simulink model "model_ekf"  (R2016a)
settings: Solver=VariableStepAuto  StartTime=0.0  StopTime=50  FixedStep=T  RelTol=1e-3
undefined symbols (not defined in the file): C, g, I, K, k1, k2, Ki, l, m, Q, sigbuilder_block, T_sens, Ts
libraries: aerolibutil x2
settings Model: Creator=Patrick  LastModifiedBy=Patrick

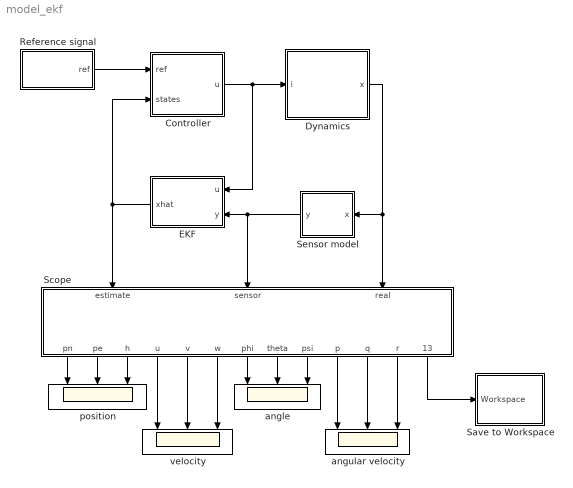
== system model_ekf ==
  Controller : Subsystem
  Dynamics : Subsystem
  EKF : Subsystem
  Reference signal : Subsystem
  Save to Workspace : Subsystem
  Scope : Subsystem
  Sensor model : Subsystem
  angle : Scope  NumInputPorts=3
  angular velocity : Scope  NumInputPorts=3
  position : Scope  NumInputPorts=3
  velocity : Scope  NumInputPorts=3
  wires:
  Sensor model/1(y) -> Scope/2(sensor), EKF/2(y)
  Reference signal/1(ref) -> Controller/1(ref)
  EKF/1(xhat) -> Scope/1(estimate), Controller/2(states)
  Dynamics/1(x) -> Scope/3(real), Sensor model/1(x)
  Controller/1(u) -> EKF/1(u), Dynamics/1(i)
  Scope/5(v) -> velocity/2
  Scope/6(w) -> velocity/3
  Scope/8(theta) -> angle/2
  Scope/9(psi) -> angle/3
  Scope/11(q) -> angular velocity/2
  Scope/10(p) -> angular velocity/1
  Scope/12(r) -> angular velocity/3
  Scope/1(pn) -> position/1
  Scope/2(pe) -> position/2
  Scope/3(h) -> position/3
  Scope/4(u) -> velocity/1
  Scope/7(phi) -> angle/1
  Scope/13(Workspace) -> Save to Workspace/1(Workspace)

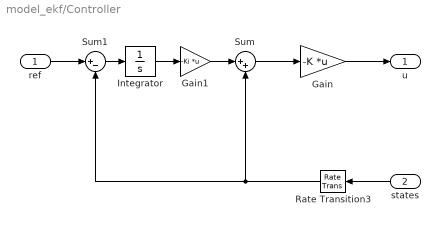
== system model_ekf/Controller ==
  ref : Inport
  states : Inport  Port=2
  Gain : Gain  Gain=-K  Multiplication=Matrix(K*u)
  Gain1 : Gain  Gain=-Ki  Multiplication=Matrix(K*u)
  Integrator : Integrator  InitialCondition=[0;0;0;0;0;0;0;0;0;0;0;0]
  Rate Transition3 : RateTransition  OutPortSampleTime=T
  Sum : Sum  Inputs=|++
  Sum1 : Sum  Inputs=|+-
  u : Outport
  wires:
  Gain1/1 -> Sum/1
  ref/1 -> Sum1/1
  Sum1/1 -> Integrator/1
  Integrator/1 -> Gain1/1
  states/1 -> Rate Transition3/1
  Sum/1 -> Gain/1
  Gain/1 -> u/1
  Rate Transition3/1 -> Sum1/2, Sum/2

== system model_ekf/Dynamics ==
  i : Inport
  Dynamics : Subsystem
  Mux : Mux
  x : Outport
  wires:
  Mux/1 -> x/1
  i/1 -> Dynamics/1(delta)
  Dynamics/1(pn pe h) -> Mux/1
  Dynamics/2(u v w) -> Mux/2
  Dynamics/3(phi theta psi) -> Mux/3
  Dynamics/4(p q r) -> Mux/4

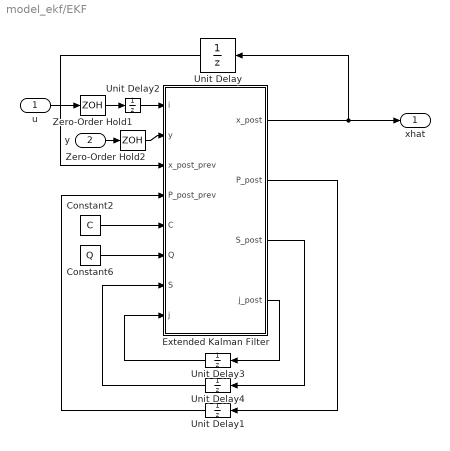
== system model_ekf/EKF ==
  u : Inport
  y : Inport  Port=2
  Constant2 : Constant  Value=C
  Constant6 : Constant  Value=Q
  Extended Kalman Filter : MATLAB Function  TreatAsAtomicUnit=on
  Unit Delay : UnitDelay  InitialCondition=[0;0;0;0;0;0;0;0;0;0;0;0]  SampleTime=Ts
  Unit Delay1 : UnitDelay  InitialCondition=zeros(12,12)  SampleTime=Ts
  Unit Delay2 : UnitDelay  InitialCondition=[0;0;0;0]  SampleTime=Ts
  Unit Delay3 : UnitDelay  InitialCondition=1  SampleTime=Ts
  Unit Delay4 : UnitDelay  InitialCondition=ones(12,1)*.004  SampleTime=Ts
  Zero-Order Hold1 : ZeroOrderHold  SampleTime=Ts
  Zero-Order Hold2 : ZeroOrderHold  SampleTime=Ts
  xhat : Outport
  wires:
  Constant2/1 -> Extended Kalman Filter/5(C)
  Constant6/1 -> Extended Kalman Filter/6(Q)
  y/1 -> Zero-Order Hold2/1
  Unit Delay/1 -> Extended Kalman Filter/3(x_post_prev)
  Unit Delay1/1 -> Extended Kalman Filter/4(P_post_prev)
  Zero-Order Hold1/1 -> Unit Delay2/1
  Extended Kalman Filter/1(x_post) -> Unit Delay/1, xhat/1
  Extended Kalman Filter/2(P_post) -> Unit Delay1/1
  Zero-Order Hold2/1 -> Extended Kalman Filter/2(y)
  u/1 -> Zero-Order Hold1/1
  Unit Delay2/1 -> Extended Kalman Filter/1(i)
  Unit Delay3/1 -> Extended Kalman Filter/8(j)
  Extended Kalman Filter/4(j_post) -> Unit Delay3/1
  Unit Delay4/1 -> Extended Kalman Filter/7(S)
  Extended Kalman Filter/3(S_post) -> Unit Delay4/1

== system model_ekf/Reference signal ==
  Mux : Mux  Inputs=12
  phi theta psi : Subsystem
  phi theta psi1 : Subsystem
  pn pe h : Subsystem
  u v w : Subsystem
  ref : Outport
  wires:
  pn pe h/1(pn) -> Mux/1
  pn pe h/2(pe) -> Mux/2
  pn pe h/3(h) -> Mux/3
  u v w/1(u) -> Mux/4
  u v w/2(v) -> Mux/5
  u v w/3(w) -> Mux/6
  phi theta psi/1(phi) -> Mux/7
  phi theta psi/2(theta) -> Mux/8
  phi theta psi/3(psi) -> Mux/9
  phi theta psi1/1(p) -> Mux/10
  phi theta psi1/2(q) -> Mux/11
  phi theta psi1/3(r) -> Mux/12
  Mux/1 -> ref/1

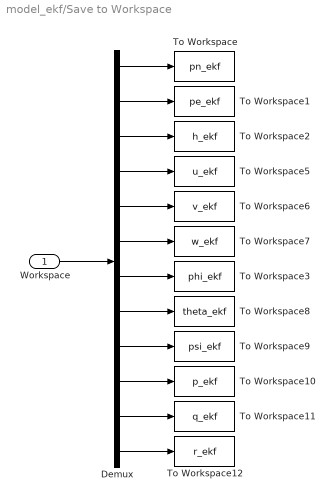
== system model_ekf/Save to Workspace ==
  Workspace : Inport
  Demux : Demux  Outputs=12
  To Workspace : ToWorkspace  VariableName=pn_ekf  SaveFormat=Timeseries  SampleTime=-1
      settings: Decimation=10
  To Workspace1 : ToWorkspace  VariableName=pe_ekf  SaveFormat=Timeseries  SampleTime=-1
      settings: Decimation=10
  To Workspace10 : ToWorkspace  VariableName=p_ekf  SaveFormat=Timeseries  SampleTime=-1
      settings: Decimation=10
  To Workspace11 : ToWorkspace  VariableName=q_ekf  SaveFormat=Timeseries  SampleTime=-1
      settings: Decimation=10
  To Workspace12 : ToWorkspace  VariableName=r_ekf  SaveFormat=Timeseries  SampleTime=-1
      settings: Decimation=10
  To Workspace2 : ToWorkspace  VariableName=h_ekf  SaveFormat=Timeseries  SampleTime=-1
      settings: Decimation=10
  To Workspace3 : ToWorkspace  VariableName=phi_ekf  SaveFormat=Timeseries  SampleTime=-1
      settings: Decimation=10
  To Workspace5 : ToWorkspace  VariableName=u_ekf  SaveFormat=Timeseries  SampleTime=-1
      settings: Decimation=10
  To Workspace6 : ToWorkspace  VariableName=v_ekf  SaveFormat=Timeseries  SampleTime=-1
      settings: Decimation=10
  To Workspace7 : ToWorkspace  VariableName=w_ekf  SaveFormat=Timeseries  SampleTime=-1
      settings: Decimation=10
  To Workspace8 : ToWorkspace  VariableName=theta_ekf  SaveFormat=Timeseries  SampleTime=-1
      settings: Decimation=10
  To Workspace9 : ToWorkspace  VariableName=psi_ekf  SaveFormat=Timeseries  SampleTime=-1
      settings: Decimation=10
  wires:
  Workspace/1 -> Demux/1
  Demux/1 -> To Workspace/1
  Demux/2 -> To Workspace1/1
  Demux/3 -> To Workspace2/1
  Demux/4 -> To Workspace5/1
  Demux/5 -> To Workspace6/1
  Demux/6 -> To Workspace7/1
  Demux/7 -> To Workspace3/1
  Demux/8 -> To Workspace8/1
  Demux/10 -> To Workspace10/1
  Demux/9 -> To Workspace9/1
  Demux/11 -> To Workspace11/1
  Demux/12 -> To Workspace12/1

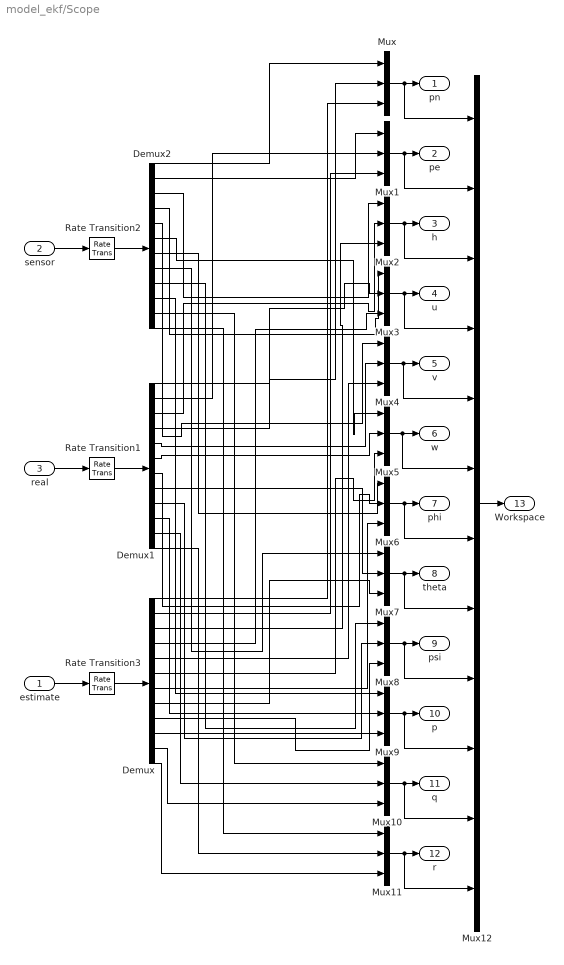
== system model_ekf/Scope ==
  estimate : Inport
  sensor : Inport  Port=2
  real : Inport  Port=3
  Demux : Demux  Outputs=12
  Demux1 : Demux  Outputs=12
  Demux2 : Demux  Outputs=12
  Mux{,1..11} (12 alike) : Mux  Inputs=3
  Mux12 : Mux  Inputs=12
  Rate Transition1 : RateTransition  OutPortSampleTime=T
  Rate Transition2 : RateTransition  OutPortSampleTime=T
  Rate Transition3 : RateTransition  OutPortSampleTime=T
  pn : Outport
  pe : Outport  Port=2
  h : Outport  Port=3
  u : Outport  Port=4
  v : Outport  Port=5
  w : Outport  Port=6
  phi : Outport  Port=7
  theta : Outport  Port=8
  psi : Outport  Port=9
  p : Outport  Port=10
  q : Outport  Port=11
  r : Outport  Port=12
  Workspace : Outport  Port=13
  wires:
  estimate/1 -> Rate Transition3/1
  real/1 -> Rate Transition1/1
  sensor/1 -> Rate Transition2/1
  Demux2/1 -> Mux/1
  Demux1/1 -> Mux/2
  Demux/1 -> Mux/3
  Demux2/2 -> Mux1/1
  Demux1/2 -> Mux1/2
  Demux/2 -> Mux1/3
  Demux2/3 -> Mux2/1
  Demux1/3 -> Mux2/2
  Demux/3 -> Mux2/3
  Mux/1 -> Mux12/1, pn/1
  Mux1/1 -> Mux12/2, pe/1
  Demux2/4 -> Mux3/1
  Demux1/4 -> Mux3/2
  Demux/4 -> Mux3/3
  Mux3/1 -> Mux12/4, u/1
  Demux2/5 -> Mux4/1
  Demux1/5 -> Mux4/2
  Demux/5 -> Mux4/3
  Mux4/1 -> Mux12/5, v/1
  Demux2/6 -> Mux5/1
  Demux1/6 -> Mux5/2
  Demux/6 -> Mux5/3
  Mux5/1 -> Mux12/6, w/1
  Mux6/1 -> Mux12/7, phi/1
  Demux2/7 -> Mux6/1
  Demux1/7 -> Mux6/2
  Demux/7 -> Mux6/3
  Mux7/1 -> Mux12/8, theta/1
  Demux2/8 -> Mux7/1
  Demux1/8 -> Mux7/2
  Demux/8 -> Mux7/3
  Mux8/1 -> Mux12/9, psi/1
  Demux2/9 -> Mux8/1
  Demux1/9 -> Mux8/2
  Demux/9 -> Mux8/3
  Mux9/1 -> Mux12/10, p/1
  Mux10/1 -> Mux12/11, q/1
  Mux11/1 -> Mux12/12, r/1
  Demux2/10 -> Mux9/1
  Demux1/10 -> Mux9/2
  Demux/10 -> Mux9/3
  Demux2/11 -> Mux10/1
  Demux1/11 -> Mux10/2
  Demux/11 -> Mux10/3
  Demux2/12 -> Mux11/1
  Demux1/12 -> Mux11/2
  Demux/12 -> Mux11/3
  Rate Transition3/1 -> Demux/1
  Rate Transition1/1 -> Demux1/1
  Rate Transition2/1 -> Demux2/1
  Mux2/1 -> Mux12/3, h/1
  Mux12/1 -> Workspace/1

== system model_ekf/Sensor model ==
  x : Inport
  Gain : Gain  Gain=2
  Subsystem : Subsystem
  Sum : Sum  Inputs=|++
  Zero-Order Hold1 : ZeroOrderHold  SampleTime=T_sens
  y : Outport
  wires:
  x/1 -> Zero-Order Hold1/1
  Zero-Order Hold1/1 -> Sum/1
  Sum/1 -> y/1
  Subsystem/1(Noise) -> Gain/1
  Gain/1 -> Sum/2

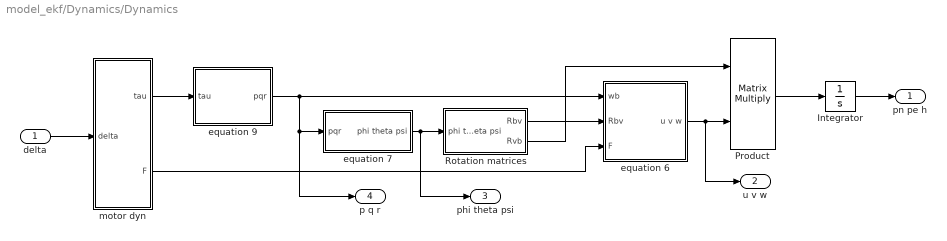
== system model_ekf/Dynamics/Dynamics ==
  delta : Inport
  Integrator : Integrator
  Product : Product  Multiplication=Matrix(*)
  Rotation matrices : Subsystem
  equation 6 : Subsystem
  equation 7 : Subsystem
  equation 9 : Subsystem
  motor dyn : Subsystem
  pn pe h : Outport
  u v w : Outport  Port=2
  phi theta psi : Outport  Port=3
  p q r : Outport  Port=4
  wires:
  Product/1 -> Integrator/1
  Rotation matrices/2(Rvb) -> Product/1
  equation 9/1(pqr) -> equation 7/1(pqr), p q r/1, equation 6/1(wb)
  equation 7/1(phi theta psi) -> Rotation matrices/1(phi theta psi), phi theta psi/1
  delta/1 -> motor dyn/1(delta)
  motor dyn/1(tau) -> equation 9/1(tau)
  equation 6/1(u v w) -> u v w/1, Product/2
  Integrator/1 -> pn pe h/1
  motor dyn/2(F) -> equation 6/3(F)
  Rotation matrices/1(Rbv) -> equation 6/2(Rbv)

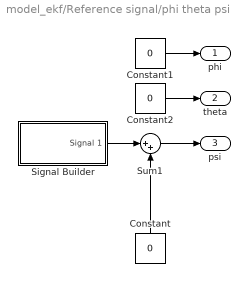
== system model_ekf/Reference signal/phi theta psi ==
  Constant : Constant  Value=0
  Constant1 : Constant  Value=0
  Constant2 : Constant  Value=0
  Signal Builder : Subsystem  Tag=STV Subsys  LoadFcn=sigbuilder_block('load');  StartFcn=sigbuilder_block('start');  StopFcn=sigbuilder_block('stop');  ClipboardFcn=sigbuilder_block('clipboard');  mask(Sigbuilder block){}
      mask help: Simulink:masks:SigbuilderBlock_MD
      mask init:
      | if ~strcmp(get_param(bdroot(gcbh),'SimulationStatus'),'stopped') tuvar = sigbuilder_block('maskInit'); end
      settings: CopyFcn=sigbuilder_block('copy');  DeleteFcn=sigbuilder_block('delete');  ModelCloseFcn=sigbuilder_block('modelClose');  PreSaveFcn=sigbuilder_block('preSave');  PauseFcn=sigbuilder_block('pause');  ContinueFcn=sigbuilder_block('continue');  NameChangeFcn=sigbuilder_block('namechange');  OpenFcn=sigbuilder_block('open',[777.75 160.5 550.5 399.75 ]);  CloseFcn=sigbuilder_block('close');
      mask Display: plot(0, 0, 100, 100,[2, 2, 32, 32, 2], [68, 8, 8, 68, 68],[32, 2], [38, 38], [32, 19, 2],[53, 60, 44], [32, 17, 17, 2],[16, 16, 31, 31]);txt = getActiveGroup(gcbh);text(2, 100, txt,'verticalAlignment', 'top');
  Sum1 : Sum  Inputs=|++
  phi : Outport
  theta : Outport  Port=2
  psi : Outport  Port=3
  wires:
  Signal Builder/1(Signal 1) -> Sum1/1
  Sum1/1 -> psi/1
  Constant1/1 -> phi/1
  Constant/1 -> Sum1/2
  Constant2/1 -> theta/1

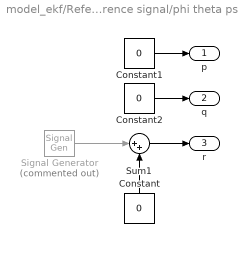
== system model_ekf/Reference signal/phi theta psi1 ==
  Constant : Constant  Value=0
  Constant1 : Constant  Value=0
  Constant2 : Constant  Value=0
  Signal Generator : SignalGenerator  Commented=on  WaveForm=square  Amplitude=.2  Frequency=.2  Units=rad/sec
  Sum1 : Sum  Inputs=|++
  p : Outport
  q : Outport  Port=2
  r : Outport  Port=3
  wires:
  Signal Generator/1 -> Sum1/1
  Sum1/1 -> r/1
  Constant/1 -> Sum1/2
  Constant1/1 -> p/1
  Constant2/1 -> q/1

== system model_ekf/Reference signal/pn pe h ==
  Constant : Constant  Value=-1
  Pulse Generator : DiscretePulseGenerator  PulseType=Time based  Period=20  PulseWidth=50
  Pulse Generator1 : DiscretePulseGenerator  PulseType=Time based  Period=20  PulseWidth=50
  Signal Generator : SignalGenerator  Commented=on  WaveForm=square  Amplitude=.2  Frequency=.2  Units=rad/sec
  Sum1 : Sum  Inputs=|++
  pn : Outport
  pe : Outport  Port=2
  h : Outport  Port=3
  wires:
  Signal Generator/1 -> Sum1/1
  Sum1/1 -> h/1
  Constant/1 -> Sum1/2
  Pulse Generator1/1 -> pe/1
  Pulse Generator/1 -> pn/1

== system model_ekf/Reference signal/u v w ==
  Constant : Constant  Value=0
  Constant1 : Constant  Value=0
  Constant2 : Constant  Value=0
  Signal Generator : SignalGenerator  Commented=on  WaveForm=square  Amplitude=.2  Frequency=.2  Units=rad/sec
  Sum1 : Sum  Inputs=|++
  u : Outport
  v : Outport  Port=2
  w : Outport  Port=3
  wires:
  Signal Generator/1 -> Sum1/1
  Sum1/1 -> w/1
  Constant/1 -> Sum1/2
  Constant1/1 -> u/1
  Constant2/1 -> v/1

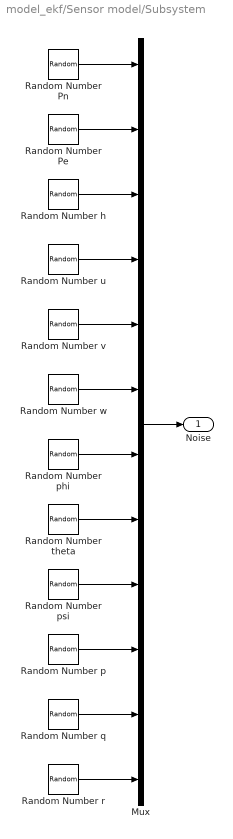
== system model_ekf/Sensor model/Subsystem ==
  Mux : Mux  Inputs=12
  Random Number Pe : RandomNumber  Variance=.001  Seed=1  SampleTime=T_sens
  Random Number Pn : RandomNumber  Variance=.001  SampleTime=T_sens
  Random Number h : RandomNumber  Variance=.001  Seed=2  SampleTime=T_sens
  Random Number p : RandomNumber  Variance=.001  Seed=9  SampleTime=T_sens
  Random Number phi : RandomNumber  Variance=.001  Seed=6  SampleTime=T_sens
  Random Number psi : RandomNumber  Variance=.001  Seed=8  SampleTime=T_sens
  Random Number q : RandomNumber  Variance=.001  Seed=10  SampleTime=T_sens
  Random Number r : RandomNumber  Variance=.001  Seed=11  SampleTime=T_sens
  Random Number theta : RandomNumber  Variance=.001  Seed=7  SampleTime=T_sens
  Random Number u : RandomNumber  Variance=.001  Seed=3  SampleTime=T_sens
  Random Number v : RandomNumber  Variance=.001  Seed=4  SampleTime=T_sens
  Random Number w : RandomNumber  Variance=.001  Seed=5  SampleTime=T_sens
  Noise : Outport
  wires:
  Random Number q/1 -> Mux/11
  Random Number r/1 -> Mux/12
  Random Number p/1 -> Mux/10
  Random Number psi/1 -> Mux/9
  Random Number phi/1 -> Mux/7
  Random Number u/1 -> Mux/4
  Random Number v/1 -> Mux/5
  Random Number w/1 -> Mux/6
  Random Number theta/1 -> Mux/8
  Random Number Pn/1 -> Mux/1
  Random Number Pe/1 -> Mux/2
  Mux/1 -> Noise/1
  Random Number h/1 -> Mux/3

== system model_ekf/Dynamics/Dynamics/Rotation matrices ==
  phi theta psi : Inport
  Rotm in euler : MATLAB Function  TreatAsAtomicUnit=on
  Transpose : Math  Operator=transpose  SaturateOnIntegerOverflow=on
  Rbv : Outport
  Rvb : Outport  Port=2
  wires:
  phi theta psi/1 -> Rotm in euler/1(alpha)
  Rotm in euler/1(Rbv) -> Rbv/1, Transpose/1
  Transpose/1 -> Rvb/1

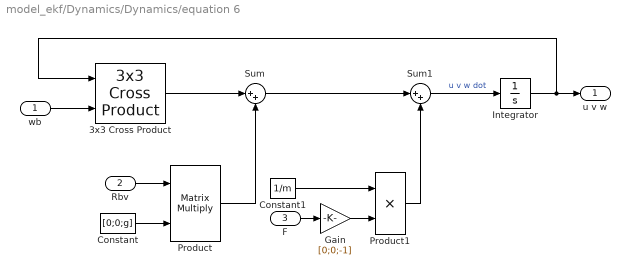
== system model_ekf/Dynamics/Dynamics/equation 6 ==
  wb : Inport
  Rbv : Inport  Port=2
  F : Inport  Port=3
  3x3 Cross Product : aerolibutil/3x3 Cross Product
  Constant : Constant  Value=[0;0;g]
  Constant1 : Constant  Value=1/m
  Gain : Gain  Gain=[0;0;-1]
  Integrator : Integrator
  Product : Product  Multiplication=Matrix(*)
  Product1 : Product
  Sum : Sum  Inputs=|++
  Sum1 : Sum  Inputs=|++
  u v w : Outport
  wires:
  3x3 Cross Product/1 -> Sum/1
  wb/1 -> 3x3 Cross Product/2
  Product/1 -> Sum/2
  Rbv/1 -> Product/1
  Constant/1 -> Product/2
  Sum/1 -> Sum1/1
  Product1/1 -> Sum1/2
  Constant1/1 -> Product1/1
  F/1 -> Gain/1
  Sum1/1 -> Integrator/1  "u v w dot"
  Integrator/1 -> 3x3 Cross Product/1, u v w/1
  Gain/1 -> Product1/2

== system model_ekf/Dynamics/Dynamics/equation 7 ==
  pqr : Inport
  Integrator : Integrator  InitialCondition=[0;0;0]
  MATLAB Function : MATLAB Function  TreatAsAtomicUnit=on
  Product : Product  Multiplication=Matrix(*)
  phi theta psi : Outport
  wires:
  MATLAB Function/1(E) -> Product/1
  pqr/1 -> Product/2
  Product/1 -> Integrator/1  "phi theta psi dot"
  Integrator/1 -> phi theta psi/1, MATLAB Function/1(alpha)

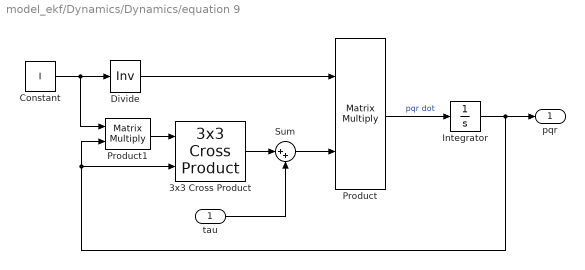
== system model_ekf/Dynamics/Dynamics/equation 9 ==
  tau : Inport
  3x3 Cross Product : aerolibutil/3x3 Cross Product
  Constant : Constant  Value=I
  Divide : Product  Inputs=/  Multiplication=Matrix(*)
  Integrator : Integrator
  Product : Product  Multiplication=Matrix(*)
  Product1 : Product  Multiplication=Matrix(*)
  Sum : Sum  Inputs=|++
  pqr : Outport
  wires:
  Constant/1 -> Product1/1, Divide/1
  Sum/1 -> Product/2
  tau/1 -> Sum/2
  3x3 Cross Product/1 -> Sum/1
  Product1/1 -> 3x3 Cross Product/1
  Divide/1 -> Product/1
  Integrator/1 -> pqr/1, 3x3 Cross Product/2, Product1/2
  Product/1 -> Integrator/1  "pqr dot"

== system model_ekf/Dynamics/Dynamics/motor dyn ==
  delta : Inport
  Force : Subsystem
  Gain : Gain  Gain=k1
  Gain1 : Gain  Gain=k2
  Torque : Subsystem
  tau : Outport
  F : Outport  Port=2
  wires:
  delta/1 -> Gain/1, Gain1/1
  Gain1/1 -> Torque/2(Tau 1234)
  Force/1(F) -> F/1
  Torque/1(tau) -> tau/1
  Gain/1 -> Torque/1(F 1234), Force/1(F 1234)

== system model_ekf/Reference signal/phi theta psi/Signal Builder ==
  Demux : Demux  Tag=STV Demux  Outputs=1
  FromWs : FromWorkspace  Tag=STV FromWs  VariableName=tuvar  SampleTime=0
      SigBuilderData=|
      | common.afterFinalStr = 'Extrapolate'
      | common.sampleTime = 0
      | dataSet.timeRange = [0 50]
      | dataSet.name = 'Group 1'
      | sbobj.Groups.Name = 'Group 1'
      | sbobj.Groups.Signals.Name = 'Signal 1'
      | sbobj.Groups.Signals.XData = [0 12.5 12.5 17.5 17.5 22.5 22.5 27.4 27.4 50]
      | sbobj.Groups.Signals.YData = [0 0 1.57079632679 1.57079632679 0 0 1.57079632679 1.57079632679 0 0]
      | sbobj.Groups.TimeRange = [0 50]
  Signal 1 : Outport  Tag=STV Outport
  wires:
  Demux/1 -> Signal 1/1
  FromWs/1 -> Demux/1

== system model_ekf/Dynamics/Dynamics/motor dyn/Force ==
  F 1234 : Inport
  Sum of Elements : Sum  Inputs=+
  F : Outport
  wires:
  F 1234/1 -> Sum of Elements/1
  Sum of Elements/1 -> F/1

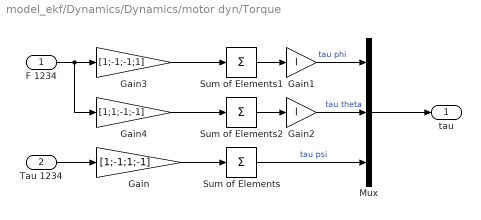
== system model_ekf/Dynamics/Dynamics/motor dyn/Torque ==
  F 1234 : Inport
  Tau 1234 : Inport  Port=2
  Gain : Gain  Gain=[1;-1;1;-1]
  Gain1 : Gain  Gain=l
  Gain2 : Gain  Gain=l
  Gain3 : Gain  Gain=[1;-1;-1;1]
  Gain4 : Gain  Gain=[1;1;-1;-1]
  Mux : Mux  Inputs=3
  Sum of Elements : Sum  Inputs=+
  Sum of Elements1 : Sum  Inputs=+
  Sum of Elements2 : Sum  Inputs=+
  tau : Outport
  wires:
  Tau 1234/1 -> Gain/1
  F 1234/1 -> Gain4/1, Gain3/1
  Gain/1 -> Sum of Elements/1
  Sum of Elements/1 -> Mux/3  "tau psi"
  Sum of Elements2/1 -> Gain2/1
  Gain2/1 -> Mux/2  "tau theta"
  Gain1/1 -> Mux/1  "tau phi"
  Mux/1 -> tau/1
  Gain3/1 -> Sum of Elements1/1
  Sum of Elements1/1 -> Gain1/1
  Gain4/1 -> Sum of Elements2/1

== matlab function model_ekf/EKF/Extended Kalman Filter ==
  data: i input; x_post output; y input; x_post_prev input; P_post_prev input; C input; Q input; S input; j input; P_post output; S_post output; j_post output
function [x_post,P_post,S_post,j_post] = fcn(i,y,x_post_prev,P_post_prev,C,Q,S,j)
coder.extrinsic('subA');
coder.extrinsic('subF');

Am = subA(x_post_prev,i);
fm = subF(x_post_prev,i);

A = zeros(12,12);
A = Am;

f = zeros(12,1);
f = fm;
%% Prediction
x_prio = f;
P_prio = A*P_post_prev*A'+Q;

%% Variance estimation
S_post = S + (j-1)*(y-x_prio).*((y-x_prio)/j);

if j>1
    R = diag(S_post)/(j-1);
else
    R = diag(S_post);
end

j_post = j+1;

%% Update
K = P_prio*C'/(C*P_prio*C'+R);
x_post = x_prio + K*(y-C*x_prio);
P_post = (eye(size(P_prio,1))-K*C)*P_prio*(eye(size(P_prio,1))-K*C)'+K*R*K';
% P_post = (eye(size(P_prio,1))-K*C)*P_prio;

== matlab function model_ekf/Dynamics/Dynamics/Rotation matrices/Rotm in euler ==
  data: alpha input; Rbv output
function Rbv = fcn(alpha)
Rbv = [1,0,0;0,cos(alpha(1)),sin(alpha(1));0,-sin(alpha(1)),cos(alpha(1))]*...
      [cos(alpha(2)),0,-sin(alpha(2));0,1,0;sin(alpha(2)),0,cos(alpha(2))]*...
      [cos(alpha(3)),sin(alpha(3)),0;-sin(alpha(3)),cos(alpha(3)),0;0,0,1];

== matlab function model_ekf/Dynamics/Dynamics/equation 7/MATLAB Function ==
  data: alpha input; E output
function E = fcn(alpha)
E = [1, sin(alpha(1))*tan(alpha(2)),cos(alpha(1))*tan(alpha(2));...
     0,               cos(alpha(1)),             -sin(alpha(1));...
     0, sin(alpha(1))/cos(alpha(2)),cos(alpha(1))/cos(alpha(2))];
